simulink model "ModelMotorSimulink"  (R2012b)
settings: Solver=ode3  StartTime=0.0  StopTime=15  FixedStep=1e-4  RelTol=1e-3
settings Model: Creator=Augusto  LastModifiedBy=Augusto

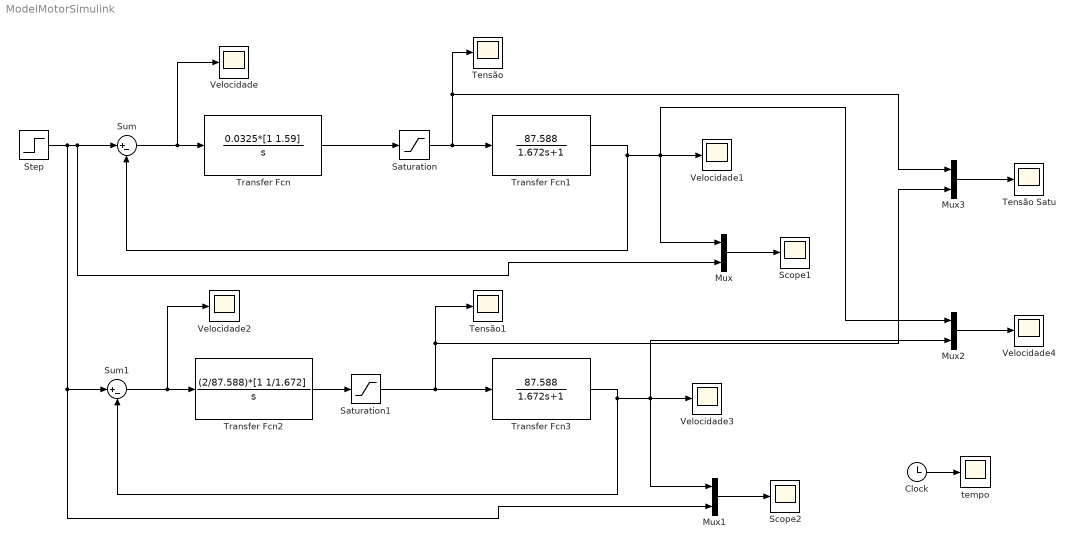
== system ModelMotorSimulink ==
  Clock : Clock
  Mux{,1..3} (4 alike) : Mux  Inputs=2
  Saturation : Saturate  UpperLimit=11.4  LowerLimit=-11.4
  Saturation1 : Saturate  UpperLimit=11.4  LowerLimit=-11.4
  Scope1 : Scope
  Scope2 : Scope
      settings: YMin=628  YMax=628  SaveName=ScopeData3
  Step : Step  Time=100  Before=600  After=-628  SampleTime=0
  Sum : Sum  Inputs=|+-
  Sum1 : Sum  Inputs=|+-
  Tensão : Scope
      settings: SaveName=ScopeData4
  Tensão Satu : Scope
      settings: SaveName=ScopeData9
  Tensão1 : Scope
      settings: SaveName=ScopeData5
  Transfer Fcn : TransferFcn  Numerator=0.0325*[1 1.59]  Denominator=[1 0]
  Transfer Fcn1 : TransferFcn  Numerator=[87.588]  Denominator=[1.672 1]
  Transfer Fcn2 : TransferFcn  Numerator=(2/87.588)*[1 1/1.672]  Denominator=[1 0]
  Transfer Fcn3 : TransferFcn  Numerator=[87.588]  Denominator=[1.672 1]
  Velocidade{,1..4} (5 alike) : Scope
      Velocidade1 settings: SaveName=ScopeData2
      Velocidade2 settings: SaveName=ScopeData6
      Velocidade3 settings: SaveName=ScopeData7
      Velocidade4 settings: TimeRange=200  YMin=-1000  YMax=1000  SaveName=ScopeData8
  tempo : Scope
      settings: Tag=Tempo  SaveName=ScopeData10
  wires:
  Mux/1 -> Scope1/1
  Sum/1 -> Velocidade/1, Transfer Fcn/1
  Transfer Fcn/1 -> Saturation/1
  Mux1/1 -> Scope2/1
  Sum1/1 -> Velocidade2/1, Transfer Fcn2/1
  Transfer Fcn2/1 -> Saturation1/1
  Transfer Fcn3/1 -> Sum1/2, Mux2/2, Mux1/1, Velocidade3/1
  Step/1 -> Sum1/1, Mux1/2, Sum/1, Mux/2
  Transfer Fcn1/1 -> Sum/2, Mux2/1, Mux/1, Velocidade1/1
  Mux2/1 -> Velocidade4/1
  Saturation/1 -> Mux3/1, Tensão/1, Transfer Fcn1/1
  Mux3/1 -> Tensão Satu/1
  Saturation1/1 -> Mux3/2, Tensão1/1, Transfer Fcn3/1
  Clock/1 -> tempo/1
